simulink model "sim_dcmotor_tf_func"  (R2021b)
settings: Solver=ode1  StartTime=0.0  StopTime=2  FixedStep=0.01  RelTol=1e-3
undefined symbols (not defined in the file): a, b, kp, z
settings Model: Creator=ASUS  LastModifiedBy=ASUS

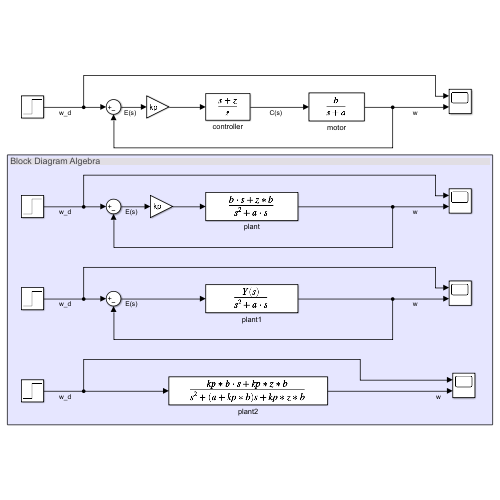
[thumbnail: Simulink's stored preview of the top-level diagram]
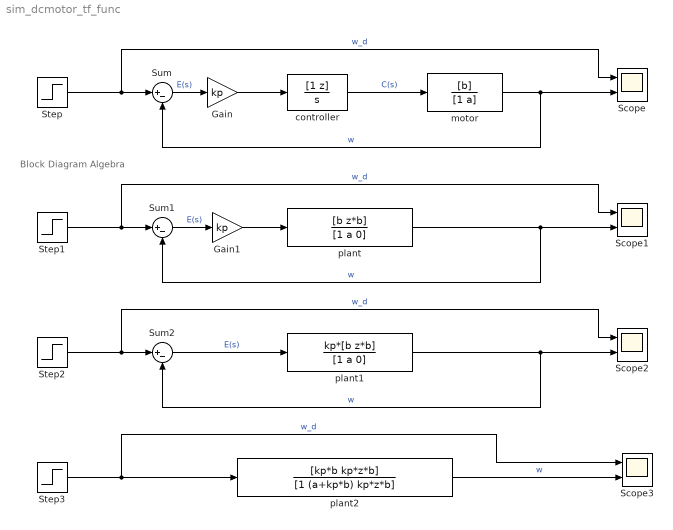
== system sim_dcmotor_tf_func ==
  note: Block Diagram Algebra
  Gain : Gain  Gain=kp
  Gain1 : Gain  Gain=kp
  Scope{,1..3} (4 alike) : Scope  NumInputPorts=2
  Step{,1..3} (4 alike) : Step  After=6  SampleTime=0
  Sum : Sum  Inputs=|+-
  Sum1 : Sum  Inputs=|+-
  Sum2 : Sum  Inputs=|+-
  controller : TransferFcn  Numerator=[1 z]  Denominator=[1 0]
  motor : TransferFcn  Numerator=[b]  Denominator=[1 a]
  plant : TransferFcn  Numerator=[b z*b]  Denominator=[1 a 0]
  plant1 : TransferFcn  Numerator=kp*[b z*b]  Denominator=[1 a 0]
  plant2 : TransferFcn  Numerator=[kp*b kp*z*b]  Denominator=[1 (a+kp*b) kp*z*b]
  wires:
  controller/1 -> motor/1  "C(s)"
  Gain/1 -> controller/1
  Sum/1 -> Gain/1  "E(s)"
  Step/1 -> Scope/1, Sum/1  "w_d"
  motor/1 -> Scope/2, Sum/2  "w"
  plant/1 -> Sum1/2, Scope1/2  "w"
  Step1/1 -> Sum1/1, Scope1/1  "w_d"
  Sum1/1 -> Gain1/1  "E(s)"
  Gain1/1 -> plant/1
  Sum2/1 -> plant1/1  "E(s)"
  Step2/1 -> Scope2/1, Sum2/1  "w_d"
  plant1/1 -> Scope2/2, Sum2/2  "w"
  plant2/1 -> Scope3/2  "w"
  Step3/1 -> plant2/1, Scope3/1  "w_d"
